simulink model "controller_template_vTST"  (Simulink 7.8)
settings: Solver=ode45  SolverMode=SingleTasking  StartTime=0.0  StopTime=20  FixedStep=Ts  RelTol=1e-3
PreLoadFcn:
  | load_waypoints
values from neighbouring files (symbols this model uses):
  Aff_pitch = [0.764669359834 -6.55628329998 -0.0099932514458 -0.411590904828 0.0133529191446 -0.0326334422872 -8.8646944178e-05 -0.00470014240893 0 0 1 0 ... (16 elements, 4x4)]    [kostas_malakies.mat]    (also in kostas_malakies2.mat)
  Aff_roll = [0.825180563081 -6.10606264808 -0.00763580464276 -0.367448917026 0.0145694646817 0.0253169520582 -6.457583527e-05 -0.00409059128644 0 0 1 0 ... (16 elements, 4x4)]    [kostas_malakies.mat]    (also in kostas_malakies2.mat; main_last.m = [Aff_roll,zeros(size(Aff_roll,1),1);zeros(1,size(Aff_roll,1))
  Aff_yaw = 0.520554464036    [kostas_malakies.mat]    (also in kostas_malakies2.mat; main.m = sysfd_yaw.a; main_last.m = sysfd_yaw.a)
  Bff_pitch = [0.235330640166  0; 6.55628329998  0; -0.000567656018985  0; -0.0435256495914  0]    [kostas_malakies.mat]    (also in kostas_malakies2.mat)
  Bff_roll = [0.174819436919  0; 6.10606264808  0; -0.000299760068643  0; -0.0270637325616  0]    [kostas_malakies.mat]    (also in kostas_malakies2.mat; main_last.m = [Bff_roll;zeros(1,size(Bff_roll,2))])
  Bff_yaw = 0.479445535964    [kostas_malakies.mat]    (also in kostas_malakies2.mat; main.m = sysfd_yaw.b; main_last.m = sysfd_yaw.b)
  Fi_XdirFF = [-0.447351940284 0 0 -1.28434394361 -4.04417159595 -1.80654990505 -1.28434394361 1 -4.04417159595 -1.80654990505 1 0 ... (536 elements, 134x4)]    [kostas_malakies.mat]    (also in kostas_malakies2.mat; matlab.mat = [-1.62441280603 -1.28434394361 -1.7723315065 -1.66810627541 )
  Fi_Yaw = [-1.14619813144 0 0]    [kostas_malakies.mat]    (also in kostas_malakies2.mat; matlab.mat = -0.284754025426)
  Fi_Ydir = [-0.466308586531 2.22044604925e-16 2.22044604925e-16 -1.46518332723 -4.54395337171 -2.00318743375 -1.46518332723 1 -4.54395337171 -2.00318743375 1 2.22044604925e-16 ... (536 elements, 134x4)]    [kostas_malakies.mat]    (also in kostas_malakies2.mat = [-0.521298425559 -2.64128186917 -15.6565978667 -8.2066553194; matlab.mat = [1 -1.9173235349 -1.46518332723 1 1 1 1 1 -1.98764774833 -1.)
  Fi_Zdir = [0 -1.80359099426e-16 0 1.4149586889 0 0 2.30859647265e-14 -5.77149118162e-15 0 0 0 0 ... (54 elements, 27x2)]    [kostas_malakies.mat]    (also in kostas_malakies2.mat = [4.30976351396 0 4.73307471514 3.80948040666 0 0 0 0.5468933; matlab.mat = [0 -9.51943523339e-14 0 1.99761158231 0 1.18992940417e-14 0 )
  g = 9.8065    [kostas_malakies.mat]    (also in kostas_malakies2.mat; load_PMModel.m = 9.81; main.m; main_last.m)
  Gi_XdirFF = [0 0.27 -0.27 0.478341621792 -6.42962779272 -1.98615606962 -0.478341621792 -0.373552567526 6.42962779272 1.98615606962 0.373552567526 0.27 ... (134 elements, 134x1)]    [kostas_malakies.mat]    (also in kostas_malakies2.mat; matlab.mat = [3.88578058619e-16 0.478341621792 -0.139455879222 -0.1159311)
  Gi_Yaw = [4.4408920985e-16 -3.14159265359 3.14159265359]    [kostas_malakies.mat]    (also in kostas_malakies2.mat = [-4.4408920985e-16 -3.14159265359 3.14159265359]; matlab.mat = 4.4408920985e-16)
  Gi_Ydir = [-2.77555756156e-16 0.27 -0.27 0.516209388722 7.06668201156 2.10835273651 -0.516209388722 -0.383863816771 -7.06668201156 -2.10835273651 0.383863816771 0.27 ... (134 elements, 134x1)]    [kostas_malakies.mat]    (also in kostas_malakies2.mat = [1.11022302463e-16 0.765579126644 531.260413192 11.754237275; matlab.mat = [0.383863816771 -0.133207088705 0.516209388722 0.38386381677)
  Gi_Zdir = [-1 -1 -1 2.22044604925e-16 -1 -1 -1 -1 1 -1 -1 -1 ... (27 elements, 27x1)]    [kostas_malakies.mat]    (also in kostas_malakies2.mat = [0.174387892495 -1 0.368373831608 3.33066907388e-16 -1 -1 -1; matlab.mat = [-2 -2 -2 1.11022302463e-15 -2 -2 -2 2 -2 -2 -2 2 ... (21 el)
  Hn_XdirFF = [-0.618529611748 0.618529611748 0.827215259158 -0.512155371354 -0.650909395739 -0.827215259158 0.930717154057 0.512155371354 0.650909395739 -0.930717154057 -1 0 ... (4464 elements, 1116x4)]    [kostas_malakies.mat]    (also in kostas_malakies2.mat; matlab.mat = [1 -0.136019433325 -0.405248495598 -0.339279056031 0 -1 0.13)
  Hn_Yaw = [1 -1 -1 1 1 -1]    [kostas_malakies.mat]    (also in kostas_malakies2.mat; matlab.mat = [1 -1])
  Hn_Ydir = [-0.642151612842 0.642151612842 0.873369621238 0.521434628645 0.668917219747 -0.873369621238 0.934789012395 -0.521434628645 -0.668917219747 -0.934789012395 -1 0 ... (4532 elements, 1133x4)]    [kostas_malakies.mat]    (also in kostas_malakies2.mat = [0.972602710123 0.0284063109089 0.559530157965 0.73050130567; matlab.mat = [0.711566553558 0.999813894311 -0.735660470031 0 0 0.5471922)
  Hn_Zdir = [-0.560552458797 -0.996815278536 -0.988320507921 0.666673243042 -1 0 -0.421994354267 -0.987440631917 -0.973284290019 -0.956170964903 -0.936236606521 0.560552458797 ... (224 elements, 112x2)]    [kostas_malakies.mat]    (also in kostas_malakies2.mat = [-0.781813705838 -0.712499731132 0.751798766698 0 -0.7286973; matlab.mat = [1 -1 -0.996815278536 -0.990718937584 -0.276007160242 0.3840)
  Kn_XdirFF = [0.373314565409 0.373314565409 0.472754204418 0.915522246067 0.951154784392 0.472754204418 0.240212330437 0.915522246067 0.951154784392 0.240212330437 0.2094 2 ... (1116 elements, 1116x1)]    [kostas_malakies.mat]    (also in kostas_malakies2.mat; matlab.mat = [0.2094 0.19132523886 0.382063154155 0.900203176458 2 0.2094)
  Kn_Yaw = [2.74088097634 2.74088097634 -2.74088097634 3.14159265359 -2.74088097634 3.14159265359]    [kostas_malakies.mat]    (also in kostas_malakies2.mat; matlab.mat = [0.0873 0.0873])
  Kn_Ydir = [0.371815875743 0.371815875743 0.451349483511 0.90366201682 0.917647772499 0.451349483511 0.24471770913 0.90366201682 0.917647772499 0.24471770913 0.2094 2 ... (1133 elements, 1133x1)]    [kostas_malakies.mat]    (also in kostas_malakies2.mat = [0.351231202126 0.997082913977 0.855763802521 0.792250278627; matlab.mat = [-0.126119149197 0.0536759032179 0.37354703421 2 2 -0.239682)
  Kn_Zdir = [0.727672356179 1.00172267683 1.00656919451 -0.471160923828 1 1 1.18526984431 1.00688561667 1.01272393898 1.01603878926 1.01572683497 -0.727672356179 ... (112 elements, 112x1)]    [kostas_malakies.mat]    (also in kostas_malakies2.mat = [0.21304012328 0.326509029469 -0.262060822346 1 0.301409884 ; matlab.mat = [1 1 1.00663007512 1.02122194908 0.632590992205 -0.384463644)
  Nc_XdirFF = [18 15 15 11 9 7 11 14 9 7 14 8 ... (134 elements, 134x1)]    [kostas_malakies.mat]    (also in kostas_malakies2.mat; matlab.mat = [14 8 7 10 8 7 10 12 10 10 12 11 ... (107 elements, 107x1)])
  Nc_Yaw = [2 2 2]    [kostas_malakies.mat]    (also in kostas_malakies2.mat; matlab.mat = 2)
  Nc_Ydir = [18 16 16 10 9 7 10 14 9 7 14 8 ... (134 elements, 134x1)]    [kostas_malakies.mat]    (also in kostas_malakies2.mat = [22 12 6 9 9 5 12 13 6 9 9 5 ... (171 elements, 171x1)]; matlab.mat = [11 8 12 15 7 9 10 13 10 14 12 7 ... (104 elements, 104x1)])
  Nc_Zdir = [6 7 3 6 3 4 4 3 6 5 3 4 ... (27 elements, 27x1)]    [kostas_malakies.mat]    (also in kostas_malakies2.mat = [4 4 3 12 5 4 3 3 4 3 3 4 ... (93 elements, 93x1)]; matlab.mat = [6 3 7 4 4 3 4 6 3 5 3 3 ... (21 elements, 21x1)])
  pitch_cmd2pitch_1stOrd = 1.42468924998    [kostas_malakies.mat]    (also in kostas_malakies2.mat)
  roll_cmd2roll_1stOrd = 1.38101661575    [kostas_malakies.mat]    (also in kostas_malakies2.mat)
  thrust_cmd2thrust_0thOrd = 0.876575459522    [kostas_malakies.mat]    (also in kostas_malakies2.mat)
  THRUST_CMD_GAIN = -0.0835    [kostas_malakies.mat]    (also in kostas_malakies2.mat; load_PMModel.m)
  Ts = 0.02    [kostas_malakies.mat]    (also in kostas_malakies2.mat; main.m; main_last.m; matlab.mat = 0.08)
  yaw_cmd2yaw_1stOrd = 2.01792090263    [kostas_malakies.mat]    (also in kostas_malakies2.mat)
  z = [-0.93079906702 -0.933865725994 -0.937557637691 -0.939011216164 -0.94143640995 -0.944628417492 -0.947235524654 -0.949601888657 -0.952827751637 -0.9567258358 -0.958320975304 -0.960991024971 ... (7988 elements, 7988x1)]    [kostas_malakies2.mat]    (also in plotDataTest.m = simout_data.signals.values(:,11))
libraries: simulink x6, Hquad_control_LIB_MPC x5
(part 1 of 2)
settings Model: Creator=janosch  LastModifiedBy=burrimi
settings DataIOCC: SaveOutput=off  SaveTime=off
settings OptimizationCC: OptimizeModelRefInitCode=on  LifeSpan=Inf
settings DebuggingCC: ParameterPrecisionLossMsg=none
settings HardwareCC: ProdIntDivRoundTo=Zero  ProdEndianess=LittleEndian  ProdHWDeviceType=Intel Pentium
settings RTWCC: SystemTargetFile=ert.tlc  TemplateMakefile=ert_default_tmf  Description=Embedded Coder  ProcessScript=ert_make_rtw_hook  CustomHeaderCode=#include <math.h>  TargetLang=C++  RTWCompilerOptimization=On
settings CodeAppCC: IgnoreCustomStorageClasses=off
settings ERTTargetCC: MultiwordLength=2048  GenerateSampleERTMain=on  ExtMode=on  ERTCustomFileTemplate=example_file_process.tlc  ConvertIfToSwitch=off  SuppressUnreachableDefaultCases=off

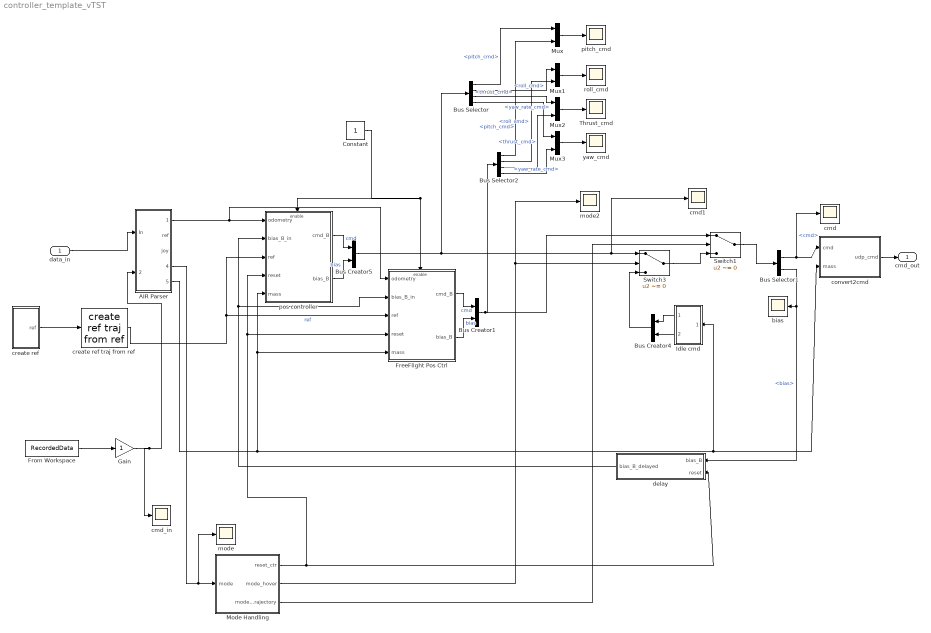
== system controller_template_vTST ==
  data_in : Inport  OutDataTypeStr=single  PortDimensions=30
  AIR Parser : Subsystem
  Bus Creator1 : BusCreator  Inputs=2
  Bus Creator4 : BusCreator  Inputs=2
  Bus Creator5 : BusCreator  Inputs=2
  Bus Selector : BusSelector  OutputSignals=cmd.pitch_cmd,cmd.roll_cmd,cmd.thrust_cmd,cmd.yaw_rate_cmd
  Bus Selector1 : BusSelector  OutputSignals=cmd,bias
  Bus Selector2 : BusSelector  OutputSignals=cmd.pitch_cmd,cmd.roll_cmd,cmd.thrust_cmd,cmd.yaw_rate_cmd
  Constant : Constant
  FreeFlight Pos Ctrl : Subsystem  AncestorBlock=Hquad_control_LIB_MPC/pos controller
  From Workspace : FromWorkspace  VariableName=RecordedData  SampleTime=0
  Gain : Gain  SampleTime=Ts
  Idle cmd : Subsystem
  Mode Handling : Subsystem
  Mux{,1..3} (4 alike) : Mux  Inputs=2
  Switch1 : Switch  Criteria=u2 ~= 0
  Switch3 : Switch  Criteria=u2 ~= 0
  Thrust_cmd : Scope
      settings: YMin=-1.3  YMax=0.1  SaveName=ScopeData18
  bias : Scope
      settings: TickLabels=on  TimeRange=40  YMin=-0.3  YMax=0.075  SaveName=ScopeData9
  cmd : Scope
      settings: YMin=-0.5  YMax=7  SaveName=ScopeData4
  cmd1 : Scope
      settings: YMin=-0.5  YMax=7  SaveName=ScopeData15
  cmd_in : Scope
      settings: YMin=-0.05  YMax=1.05  SaveName=ScopeData16
  convert2cmd : Subsystem
  create ref : Subsystem  AncestorBlock=Hquad_control_LIB_LQRI/create ref
  create ref traj from ref : Hquad_control_LIB_MPC/create ref traj from ref
  delay : Subsystem
  mode : Scope
      settings: YMin=0  YMax=6  SaveName=ScopeData6
  mode2 : Scope
      settings: YMin=0  YMax=6  SaveName=ScopeData14
  pitch_cmd : Scope
      settings: YMin=-0.375  YMax=0.1  SaveName=ScopeData13
  pos controller : Subsystem  AncestorBlock=Hquad_control_LIB_MPC/pos controller
  roll_cmd : Scope
      settings: YMin=-0.275  YMax=0.125  SaveName=ScopeData17
  yaw_cmd : Scope
      settings: YMin=-0.025  YMax=0.475  SaveName=ScopeData19
  cmd_out : Outport  PortDimensions=4
  wires:
  Mode Handling/1(reset_ctr) -> delay/2(reset), pos controller/4(reset), FreeFlight Pos Ctrl/4(reset)
  Mode Handling/2(mode_hover) -> Switch3/2, mode2/1
  AIR Parser/4(mode) -> mode/1, Mode Handling/1(mode)
  Bus Creator5/1 -> Switch3/1, cmd1/1, Bus Selector/1
  pos controller/1(cmd_B) -> Bus Creator5/1  "cmd"
  pos controller/2(bias_B) -> Bus Creator5/2  "bias"
  Bus Selector1/1 -> convert2cmd/1(cmd), cmd/1  "<cmd>"
  Bus Selector1/2 -> bias/1, delay/1(bias_B)  "<bias>"
  delay/1(bias_B_delayed) -> pos controller/2(bias_B_in), FreeFlight Pos Ctrl/2(bias_B_in)
  convert2cmd/1(udp_cmd) -> cmd_out/1
  data_in/1 -> AIR Parser/1(In)
  Idle cmd/1(cmd) -> Bus Creator4/1
  Idle cmd/2(bias) -> Bus Creator4/2
  Bus Creator4/1 -> Switch3/3
  AIR Parser/1(odometry) -> pos controller/1(odometry), FreeFlight Pos Ctrl/1(odometry)
  Switch3/1 -> Switch1/3
  Switch1/1 -> Bus Selector1/1
  Mode Handling/3(mode_trajectory) -> Switch1/2
  AIR Parser/5(mass) -> Idle cmd/1(mass), convert2cmd/2(mass), pos controller/5(mass), FreeFlight Pos Ctrl/5(mass)
  create ref traj from ref/1 -> pos controller/3(ref), FreeFlight Pos Ctrl/3(ref)  "ref"
  Bus Creator1/1 -> Switch1/1, Bus Selector2/1
  FreeFlight Pos Ctrl/1(cmd_B) -> Bus Creator1/1  "cmd"
  FreeFlight Pos Ctrl/2(bias_B) -> Bus Creator1/2  "bias"
  From Workspace/1 -> Gain/1
  Gain/1 -> AIR Parser/2(Recorded), cmd_in/1
  Constant/1 -> pos controller/Enable, FreeFlight Pos Ctrl/Enable
  Bus Selector/1 -> Mux/1  "<pitch_cmd>"
  Mux/1 -> pitch_cmd/1
  create ref/1(ref) -> create ref traj from ref/1
  Mux1/1 -> roll_cmd/1
  Mux2/1 -> Thrust_cmd/1
  Mux3/1 -> yaw_cmd/1
  Bus Selector/2 -> Mux1/1  "<roll_cmd>"
  Bus Selector/3 -> Mux2/1  "<thrust_cmd>"
  Bus Selector/4 -> Mux3/1  "<yaw_rate_cmd>"
  Bus Selector2/2 -> Mux1/2  "<roll_cmd>"
  Bus Selector2/3 -> Mux2/2  "<thrust_cmd>"
  Bus Selector2/4 -> Mux3/2  "<yaw_rate_cmd>"
  Bus Selector2/1 -> Mux/2  "<pitch_cmd>"

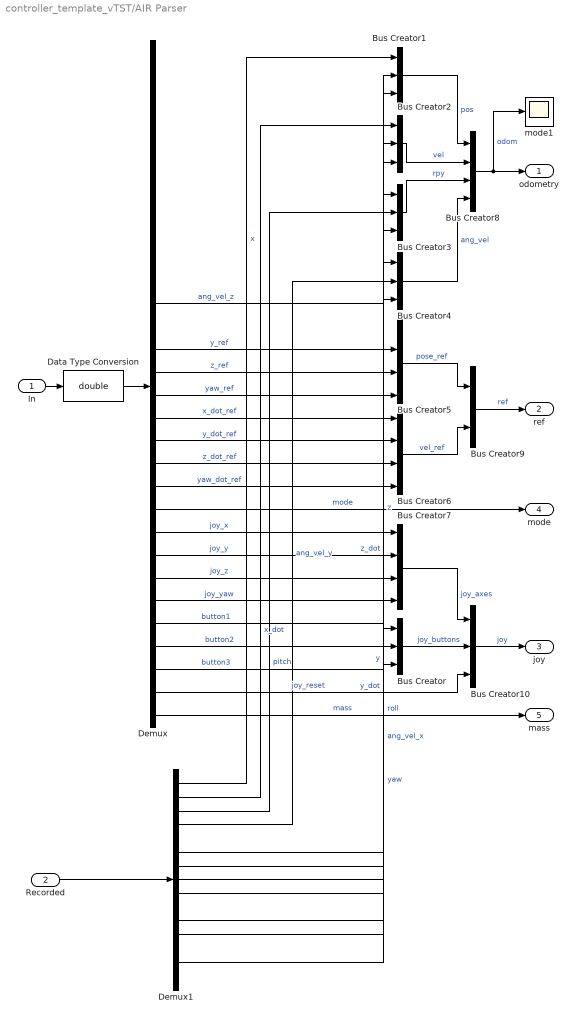
== system controller_template_vTST/AIR Parser ==
  In : Inport
  Recorded : Inport  Port=2
  Bus Creator{,1..4,10} (6 alike) : BusCreator  Inputs=3
  Bus Creator{5..8} (4 alike) : BusCreator
  Bus Creator9 : BusCreator  Inputs=2
  Data Type Conversion : DataTypeConversion  OutDataTypeStr=double
  Demux : Demux  Outputs=30
  Demux1 : Demux  Outputs=15
  mode1 : Scope
      settings: YMin=0  YMax=6  SaveName=ScopeData7
  odometry : Outport
  ref : Outport  Port=2
  joy : Outport  Port=3
  mode : Outport  Port=4
  mass : Outport  Port=5
  wires:
  In/1 -> Data Type Conversion/1
  Data Type Conversion/1 -> Demux/1
  Demux/15 -> Bus Creator5/3  "z_ref"
  Demux/14 -> Bus Creator5/2  "y_ref"
  Demux/16 -> Bus Creator5/4  "yaw_ref"
  Demux/19 -> Bus Creator6/3  "z_dot_ref"
  Demux/18 -> Bus Creator6/2  "y_dot_ref"
  Demux/17 -> Bus Creator6/1  "x_dot_ref"
  Demux/20 -> Bus Creator6/4  "yaw_dot_ref"
  Demux/12 -> Bus Creator4/3  "ang_vel_z"
  Demux/21 -> mode/1  "mode"
  Bus Creator5/1 -> Bus Creator9/1  "pose_ref"
  Bus Creator6/1 -> Bus Creator9/2  "vel_ref"
  Demux/22 -> Bus Creator7/1  "joy_x"
  Demux/23 -> Bus Creator7/2  "joy_y"
  Demux/24 -> Bus Creator7/3  "joy_z"
  Demux/25 -> Bus Creator7/4  "joy_yaw"
  Bus Creator7/1 -> Bus Creator10/1  "joy_axes"
  Demux/26 -> Bus Creator/1  "button1"
  Demux/28 -> Bus Creator/3  "button3"
  Demux/27 -> Bus Creator/2  "button2"
  Bus Creator/1 -> Bus Creator10/2  "joy_buttons"
  Bus Creator4/1 -> Bus Creator8/4  "ang_vel"
  Bus Creator3/1 -> Bus Creator8/3  "rpy"
  Bus Creator2/1 -> Bus Creator8/2  "vel"
  Bus Creator1/1 -> Bus Creator8/1  "pos"
  Demux/29 -> Bus Creator10/3  "joy_reset"
  Bus Creator10/1 -> joy/1  "joy"
  Bus Creator9/1 -> ref/1  "ref"
  Bus Creator8/1 -> odometry/1, mode1/1  "odom"
  Demux/30 -> mass/1  "mass"
  Recorded/1 -> Demux1/1
  Demux1/1 -> Bus Creator1/1  "x"
  Demux1/2 -> Bus Creator2/1  "x_dot"
  Demux1/3 -> Bus Creator3/2  "pitch"
  Demux1/4 -> Bus Creator4/2  "ang_vel_y"
  Demux1/7 -> Bus Creator2/2  "y_dot"
  Demux1/8 -> Bus Creator3/1  "roll"
  Demux1/9 -> Bus Creator4/1  "ang_vel_x"
  Demux1/12 -> Bus Creator2/3  "z_dot"
  Demux1/6 -> Bus Creator1/2  "y"
  Demux1/11 -> Bus Creator1/3  "z"
  Demux1/14 -> Bus Creator3/3  "yaw"

== system controller_template_vTST/FreeFlight Pos Ctrl ==
  odometry : Inport
  bias_B_in : Inport  Port=2
  ref : Inport  Port=3
  reset : Inport  Port=4
  mass : Inport  Port=5
  Enable : EnablePort  StatesWhenEnabling=reset
  MAIN CONTROL LOOP1 : Subsystem  Priority=2  AncestorBlock=Hquad_control_LIB_MPC/MAIN CONTROL LOOP  TreatAsAtomicUnit=on
  get ref from vector : Hquad_control_LIB_MPC/pos controller/get ref from vector
  rotate to world frame : Hquad_control_LIB_MPC/rotate to world frame  Priority=1
  view & log signals : Subsystem  AncestorBlock=Hquad_control_LIB_MPC/view & log signals
  cmd_B : Outport
  bias_B : Outport  Port=2
  wires:
  mass/1 -> MAIN CONTROL LOOP1/5(mass)
  bias_B_in/1 -> rotate to world frame/2
  rotate to world frame/2 -> MAIN CONTROL LOOP1/2(bias_W)
  rotate to world frame/1 -> MAIN CONTROL LOOP1/1(odometry), view & log signals/1(odometry)
  ref/1 -> get ref from vector/1
  reset/1 -> MAIN CONTROL LOOP1/4(reset)
  odometry/1 -> rotate to world frame/1
  get ref from vector/1 -> MAIN CONTROL LOOP1/3(ref), view & log signals/2(ref)
  MAIN CONTROL LOOP1/1(cmd_W) -> view & log signals/3(cmd), cmd_B/1
  MAIN CONTROL LOOP1/2(bias_W_out) -> view & log signals/4(bias), bias_B/1

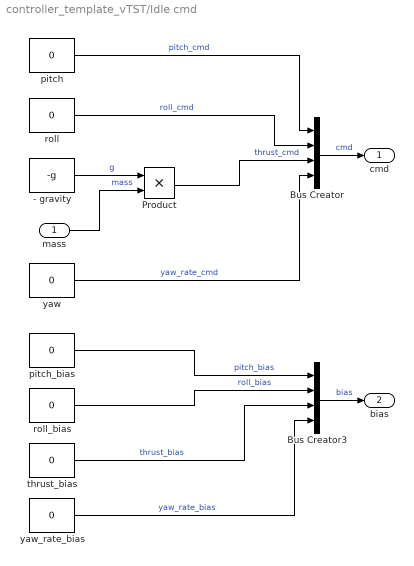
== system controller_template_vTST/Idle cmd ==
  mass : Inport  OutDataTypeStr=double
  - gravity : Constant  Value=-g
  Bus Creator : BusCreator
  Bus Creator3 : BusCreator
  Product : Product  RndMeth=Zero
  pitch : Constant  Value=0
  pitch_bias : Constant  Value=0
  roll : Constant  Value=0
  roll_bias : Constant  Value=0
  thrust_bias : Constant  Value=0
  yaw : Constant  Value=0
  yaw_rate_bias : Constant  Value=0
  cmd : Outport
  bias : Outport  Port=2
  wires:
  roll/1 -> Bus Creator/2  "roll_cmd"
  pitch/1 -> Bus Creator/1  "pitch_cmd"
  Bus Creator/1 -> cmd/1  "cmd"
  yaw/1 -> Bus Creator/4  "yaw_rate_cmd"
  pitch_bias/1 -> Bus Creator3/1  "pitch_bias"
  roll_bias/1 -> Bus Creator3/2  "roll_bias"
  thrust_bias/1 -> Bus Creator3/3  "thrust_bias"
  yaw_rate_bias/1 -> Bus Creator3/4  "yaw_rate_bias"
  Bus Creator3/1 -> bias/1  "bias"
  - gravity/1 -> Product/1  "g"
  Product/1 -> Bus Creator/3  "thrust_cmd"
  mass/1 -> Product/2  "mass"

== system controller_template_vTST/Mode Handling ==
  mode : Inport
  Constant1 : Constant
  Constant2 : Constant  Value=0
  Multiport Switch : MultiPortSwitch  DataPortOrder=Specify indices  Inputs=2  DataPortIndices={[1,2,3],0}  zeroidx=off
  Multiport Switch1 : MultiPortSwitch  DataPortOrder=Specify indices  Inputs=2  DataPortIndices={[10],0}  zeroidx=off
  Multiport Switch2 : MultiPortSwitch  DataPortOrder=Specify indices  Inputs=2  DataPortIndices={[4],0}  zeroidx=off
  reset_ctr : Outport
  mode_hover : Outport  Port=2
  mode_trajectory : Outport  Port=3
  wires:
  Constant1/1 -> Multiport Switch/2, Multiport Switch1/2, Multiport Switch2/2
  Constant2/1 -> Multiport Switch/3, Multiport Switch1/3, Multiport Switch2/3
  Multiport Switch1/1 -> reset_ctr/1
  mode/1 -> Multiport Switch/1, Multiport Switch1/1, Multiport Switch2/1
  Multiport Switch/1 -> mode_hover/1
  Multiport Switch2/1 -> mode_trajectory/1

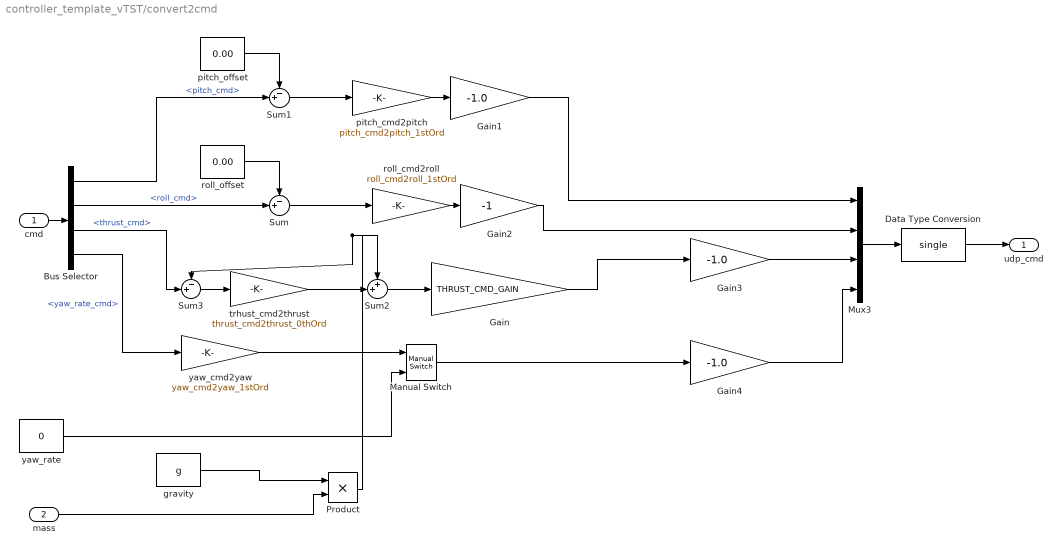
== system controller_template_vTST/convert2cmd ==
  cmd : Inport
  mass : Inport  Port=2
  Bus Selector : BusSelector  OutputSignals=pitch_cmd,roll_cmd,thrust_cmd,yaw_rate_cmd
  Data Type Conversion : DataTypeConversion  OutDataTypeStr=single
  Gain : Gain  Gain=THRUST_CMD_GAIN
  Gain1 : Gain  Gain=-1.0
  Gain2 : Gain  Gain=-1
  Gain3 : Gain  Gain=-1.0
  Gain4 : Gain  Gain=-1.0
  Manual Switch : simulink/Signal Routing/Manual Switch  sw=1  action=0  varsize=off
  Mux3 : Mux
  Product : Product  RndMeth=Zero
  Sum : Sum  Inputs=-+|
  Sum1 : Sum  Inputs=-+|
  Sum2 : Sum  Inputs=++|
  Sum3 : Sum  Inputs=-+|
  gravity : Constant  Value=g
  pitch_cmd2pitch : Gain  Gain=pitch_cmd2pitch_1stOrd
  pitch_offset : Constant  Value=0.00
  roll_cmd2roll : Gain  Gain=roll_cmd2roll_1stOrd
  roll_offset : Constant  Value=0.00
  trhust_cmd2thrust : Gain  Gain=thrust_cmd2thrust_0thOrd
  yaw_cmd2yaw : Gain  Gain=yaw_cmd2yaw_1stOrd
  yaw_rate : Constant  Value=0
  udp_cmd : Outport
  wires:
  pitch_cmd2pitch/1 -> Gain1/1
  Bus Selector/2 -> Sum/2  "<roll_cmd>"
  Sum/1 -> roll_cmd2roll/1
  roll_offset/1 -> Sum/1
  Gain4/1 -> Mux3/4
  Gain3/1 -> Mux3/3
  Gain2/1 -> Mux3/2
  Gain/1 -> Gain3/1
  Gain1/1 -> Mux3/1
  pitch_offset/1 -> Sum1/1
  Sum1/1 -> pitch_cmd2pitch/1
  Mux3/1 -> Data Type Conversion/1
  Data Type Conversion/1 -> udp_cmd/1
  Product/1 -> Sum2/1, Sum3/1
  Sum2/1 -> Gain/1
  Manual Switch/1 -> Gain4/1
  yaw_rate/1 -> Manual Switch/2
  cmd/1 -> Bus Selector/1
  Bus Selector/1 -> Sum1/2  "<pitch_cmd>"
  yaw_cmd2yaw/1 -> Manual Switch/1
  trhust_cmd2thrust/1 -> Sum2/2
  roll_cmd2roll/1 -> Gain2/1
  Bus Selector/3 -> Sum3/2  "<thrust_cmd>"
  Sum3/1 -> trhust_cmd2thrust/1
  Bus Selector/4 -> yaw_cmd2yaw/1  "<yaw_rate_cmd>"
  gravity/1 -> Product/1
  mass/1 -> Product/2

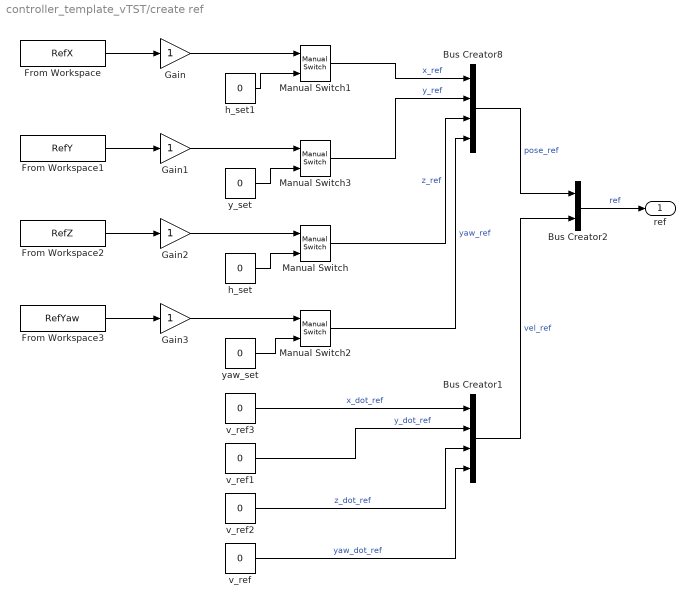
== system controller_template_vTST/create ref ==
  Bus Creator1 : BusCreator
  Bus Creator2 : BusCreator  Inputs=2
  Bus Creator8 : BusCreator
  From Workspace : FromWorkspace  VariableName=RefX  SampleTime=0
  From Workspace1 : FromWorkspace  VariableName=RefY  SampleTime=0
  From Workspace2 : FromWorkspace  VariableName=RefZ  SampleTime=0
  From Workspace3 : FromWorkspace  VariableName=RefYaw  SampleTime=0
  Gain{,1..3} (4 alike) : Gain  SampleTime=Ts
  Manual Switch{,1..3} (4 alike) : simulink/Signal Routing/Manual Switch  sw=1  action=0  varsize=off
  h_set : Constant  Value=0  OutDataTypeStr=double  SampleTime=-1
  h_set1 : Constant  Value=0  OutDataTypeStr=double  SampleTime=-1
  v_ref{,1..3} (4 alike) : Constant  Value=0  OutDataTypeStr=double  SampleTime=-1
  y_set : Constant  Value=0  OutDataTypeStr=double  SampleTime=-1
  "yaw_set  " : Constant  Value=0  OutDataTypeStr=double  SampleTime=-1
  ref : Outport
  wires:
  Gain3/1 -> Manual Switch2/1
  "yaw_set  "/1 -> Manual Switch2/2
  h_set/1 -> Manual Switch/2
  Gain2/1 -> Manual Switch/1
  Gain1/1 -> Manual Switch3/1
  y_set/1 -> Manual Switch3/2
  h_set1/1 -> Manual Switch1/2
  Bus Creator2/1 -> ref/1  "ref"
  Bus Creator8/1 -> Bus Creator2/1  "pose_ref"
  Bus Creator1/1 -> Bus Creator2/2  "vel_ref"
  Manual Switch1/1 -> Bus Creator8/1  "x_ref"
  Manual Switch3/1 -> Bus Creator8/2  "y_ref"
  Manual Switch2/1 -> Bus Creator8/4  "yaw_ref"
  Manual Switch/1 -> Bus Creator8/3  "z_ref"
  v_ref/1 -> Bus Creator1/4  "yaw_dot_ref"
  v_ref3/1 -> Bus Creator1/1  "x_dot_ref"
  v_ref1/1 -> Bus Creator1/2  "y_dot_ref"
  v_ref2/1 -> Bus Creator1/3  "z_dot_ref"
  Gain/1 -> Manual Switch1/1
  From Workspace/1 -> Gain/1
  From Workspace1/1 -> Gain1/1
  From Workspace2/1 -> Gain2/1
  From Workspace3/1 -> Gain3/1

== system controller_template_vTST/delay ==
  bias_B : Inport
  reset : Inport  Port=2
  Bus Creator1 : BusCreator
  Demux1 : Demux
  delay bias : simulink/Additional Math & Discrete/Additional Discrete/Unit Delay Resettable  vinit=0.0  tsamp=-1
  bias_B_delayed : Outport
  wires:
  Demux1/1 -> Bus Creator1/1  "pitch_bias"
  Demux1/2 -> Bus Creator1/2  "roll_bias"
  Demux1/3 -> Bus Creator1/3  "thrust_bias"
  Demux1/4 -> Bus Creator1/4  "yaw_rate_bias"
  delay bias/1 -> Demux1/1
  bias_B/1 -> delay bias/1
  reset/1 -> delay bias/2
  Bus Creator1/1 -> bias_B_delayed/1

== system controller_template_vTST/pos controller ==
  odometry : Inport
  bias_B_in : Inport  Port=2
  ref : Inport  Port=3
  reset : Inport  Port=4
  mass : Inport  Port=5
  Enable : EnablePort  StatesWhenEnabling=reset
  MAIN CONTROL LOOP1 : Hquad_control_LIB_MPC/MAIN CONTROL LOOP  Priority=2
  get ref from vector : Subsystem
  mode1 : Scope
      settings: YMin=0  YMax=6  SaveName=ScopeData12
  rotate to world frame : Hquad_control_LIB_MPC/rotate to world frame  Priority=1
  view & log signals : Subsystem  AncestorBlock=Hquad_control_LIB_MPC/view & log signals
  cmd_B : Outport
  bias_B : Outport  Port=2
  wires:
  MAIN CONTROL LOOP1/1 -> view & log signals/3(cmd), cmd_B/1
  odometry/1 -> rotate to world frame/1, view & log signals/1(odometry)
  reset/1 -> MAIN CONTROL LOOP1/4
  ref/1 -> get ref from vector/1(X_ref), MAIN CONTROL LOOP1/3
  get ref from vector/1(ref) -> view & log signals/2(ref), mode1/1
  rotate to world frame/1 -> MAIN CONTROL LOOP1/1
  MAIN CONTROL LOOP1/2 -> view & log signals/4(bias), bias_B/1
  rotate to world frame/2 -> MAIN CONTROL LOOP1/2
  bias_B_in/1 -> rotate to world frame/2
  mass/1 -> MAIN CONTROL LOOP1/5

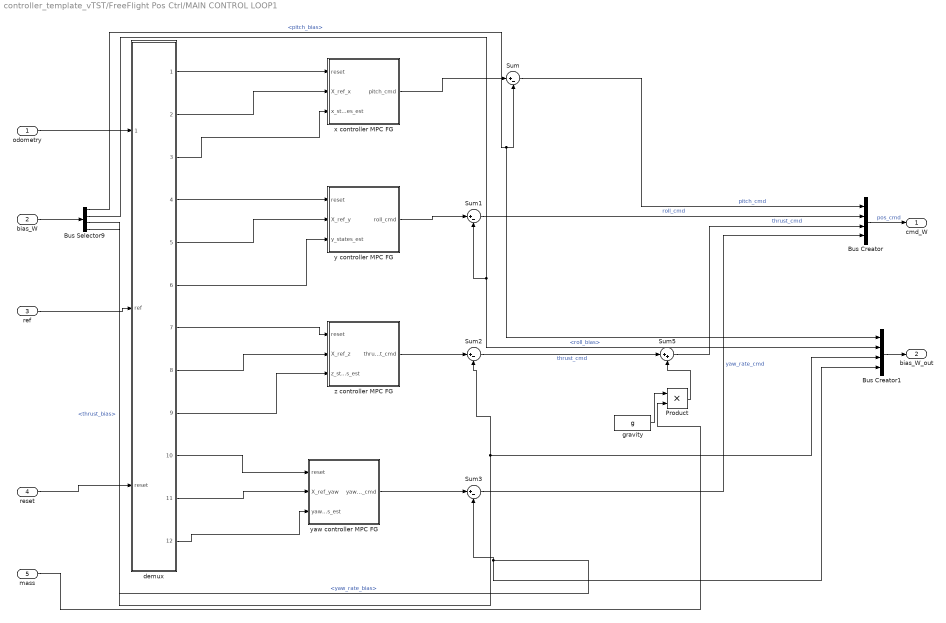
== system controller_template_vTST/FreeFlight Pos Ctrl/MAIN CONTROL LOOP1 ==
  odometry : Inport
  bias_W : Inport  Port=2
  ref : Inport  Port=3
  reset : Inport  Port=4
  mass : Inport  Port=5
  Bus Creator : BusCreator
  Bus Creator1 : BusCreator
  Bus Selector9 : BusSelector  OutputSignals=pitch_bias,roll_bias,thrust_bias,yaw_rate_bias
  Product : Product  RndMeth=Zero
  Sum{,1..3} (4 alike) : Sum  Inputs=|+-
  Sum5 : Sum  Inputs=|++
  demux : Subsystem
  gravity : Constant  Value=g
  "x controller MPC FG  " : Subsystem  AncestorBlock=Hquad_control_LIB_MPC/x controller MPC FG
  y controller MPC FG : Subsystem  AncestorBlock=Hquad_control_LIB_MPC/y controller MPC FG
  yaw controller MPC FG : Subsystem  AncestorBlock=Hquad_control_LIB_MPC/yaw controller MPC FG
  z controller MPC FG : Subsystem  AncestorBlock=Hquad_control_LIB_MPC/z controller MPC FG
  cmd_W : Outport
  bias_W_out : Outport  Port=2
  wires:
  Bus Selector9/4 -> Sum3/2, Bus Creator1/4  "<yaw_rate_bias>"
  Sum3/1 -> Bus Creator/4  "yaw_rate_cmd"
  Bus Selector9/3 -> Sum2/2, Bus Creator1/3  "<thrust_bias>"
  Bus Selector9/1 -> Sum/2, Bus Creator1/1  "<pitch_bias>"
  Bus Selector9/2 -> Bus Creator1/2, Sum1/2  "<roll_bias>"
  bias_W/1 -> Bus Selector9/1
  Sum5/1 -> Bus Creator/3  "thrust_cmd"
  Bus Creator1/1 -> bias_W_out/1
  Sum2/1 -> Sum5/1  "thrust_cmd"
  Sum1/1 -> Bus Creator/2  "roll_cmd"
  Sum/1 -> Bus Creator/1  "pitch_cmd"
  odometry/1 -> demux/1(odometry)
  ref/1 -> demux/2(ref)
  reset/1 -> demux/3(reset)
  demux/1(reset1) -> "x controller MPC FG  "/1(reset)
  demux/4(reset2) -> y controller MPC FG/1(reset)
  demux/7(reset3) -> z controller MPC FG/1(reset)
  demux/10(reset4) -> yaw controller MPC FG/1(reset)
  Bus Creator/1 -> cmd_W/1  "pos_cmd"
  mass/1 -> Product/2
  Product/1 -> Sum5/2
  gravity/1 -> Product/1
  "x controller MPC FG  "/1("pitch_cmd   ") -> Sum/1
  y controller MPC FG/1(roll_cmd) -> Sum1/1
  z controller MPC FG/1(thrust_cmd) -> Sum2/1
  yaw controller MPC FG/1(yaw_rate_cmd) -> Sum3/1
  demux/2(X_ref_x) -> "x controller MPC FG  "/2("X_ref_x  ")
  demux/3(x_states) -> "x controller MPC FG  "/3("x_states_est  ")
  demux/5(X_ref_y) -> y controller MPC FG/2("X_ref_y  ")
  demux/8(X_ref_z) -> z controller MPC FG/2(X_ref_z)
  demux/9(z_states) -> z controller MPC FG/3("z_states_est  ")
  demux/11(X_ref_yaw) -> yaw controller MPC FG/2(X_ref_yaw)
  demux/12(yaw_states) -> yaw controller MPC FG/3("yaw_states_est  ")
  demux/6(y_states) -> y controller MPC FG/3("y_states_est  ")

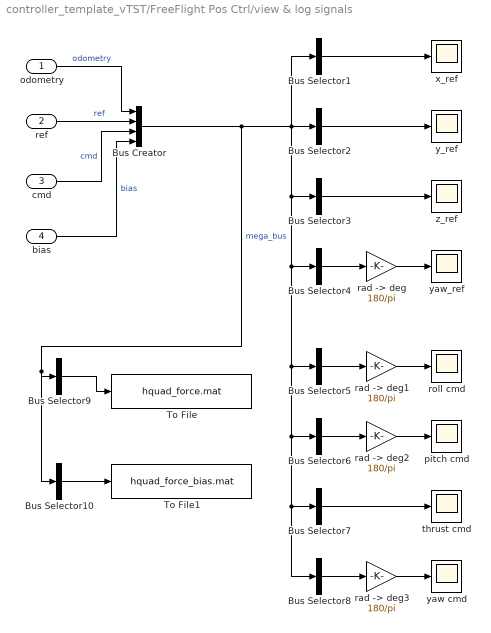
== system controller_template_vTST/FreeFlight Pos Ctrl/view & log signals ==
  odometry : Inport
  ref : Inport  Port=2
  cmd : Inport  Port=3
  bias : Inport  Port=4
  Bus Creator : BusCreator
  Bus Selector1 : BusSelector  OutputSignals=odometry.pos.x,odometry.vel.x_dot,ref.pose_ref.x_ref,ref.vel_ref.x_dot_ref  OutputAsBus=on
  Bus Selector10 : BusSelector  OutputSignals=bias.pitch_bias,bias.roll_bias,bias.thrust_bias,bias.yaw_rate_bias  OutputAsBus=on
  Bus Selector2 : BusSelector  OutputSignals=odometry.pos.y,odometry.vel.y_dot,ref.pose_ref.y_ref,ref.vel_ref.y_dot_ref  OutputAsBus=on
  Bus Selector3 : BusSelector  OutputSignals=odometry.pos.z,odometry.vel.z_dot,ref.pose_ref.z_ref,ref.vel_ref.z_dot_ref  OutputAsBus=on
  Bus Selector4 : BusSelector  OutputSignals=odometry.rpy.yaw,odometry.ang_vel.ang_vel_z,ref.pose_ref.yaw_ref,ref.vel_ref.yaw_dot_ref  OutputAsBus=on
  Bus Selector5 : BusSelector  OutputSignals=odometry.rpy.roll,odometry.ang_vel.ang_vel_x,cmd.roll_cmd  OutputAsBus=on
  Bus Selector6 : BusSelector  OutputSignals=odometry.rpy.pitch,odometry.ang_vel.ang_vel_y,cmd.pitch_cmd  OutputAsBus=on
  Bus Selector7 : BusSelector  OutputSignals=odometry.pos.z,ref.pose_ref.z_ref,cmd.thrust_cmd  OutputAsBus=on
  Bus Selector8 : BusSelector  OutputSignals=odometry.rpy.yaw,odometry.ang_vel.ang_vel_z,cmd.yaw_rate_cmd  OutputAsBus=on
  Bus Selector9 : BusSelector  OutputSignals=odometry.pos.x,odometry.vel.x_dot,odometry.rpy.pitch,ref.pose_ref.x_ref,cmd.pitch_cmd,odometry.pos.y,odometry.vel.y_dot,odometry.rpy.roll,ref.pose_ref.y_ref,cmd.roll_cmd,odometry.pos.z,odometry.vel.z_dot,ref.pose_ref.z_ref,cmd.thrust_cmd,odometry.rpy.yaw,odometry.ang_vel.ang_vel_z,ref.pose_ref.yaw_ref,cmd.yaw_rate_cmd  OutputAsBus=on
  To File : ToFile  Filename=hquad_force.mat  MatrixName=hquad_force
  To File1 : ToFile  Filename=hquad_force_bias.mat  MatrixName=hquad_force_bias
  pitch cmd : Scope
      settings: YMin=-15  YMax=15  SaveName=ScopeData2
  rad -> deg{,1..3} (4 alike) : Gain  Gain=180/pi
  roll cmd : Scope
      settings: YMin=-100  YMax=100
  thrust cmd : Scope
      settings: YMin=-3  YMax=3  SaveName=ScopeData11
  x_ref : Scope
      settings: YMin=-1.5  YMax=1.5  SaveName=ScopeData3
  y_ref : Scope
      settings: TimeRange=40  YMin=-0.75  YMax=2.75
  yaw cmd : Scope
      settings: YMin=-60  YMax=60  SaveName=ScopeData10
  yaw_ref : Scope
      settings: TimeRange=39.996  YMin=-190  YMax=190  SaveName=ScopeData8
  z_ref : Scope
      settings: TimeRange=40  YMin=-21  YMax=1  SaveName=ScopeData5
  wires:
  bias/1 -> Bus Creator/4  "bias"
  Bus Selector8/1 -> "rad -> deg3"/1
  Bus Selector6/1 -> "rad -> deg2"/1
  Bus Selector5/1 -> "rad -> deg1"/1
  Bus Selector7/1 -> thrust cmd/1
  Bus Selector4/1 -> "rad -> deg"/1
  Bus Selector3/1 -> z_ref/1
  Bus Selector2/1 -> y_ref/1
  Bus Selector1/1 -> x_ref/1
  Bus Creator/1 -> Bus Selector8/1, Bus Selector7/1, Bus Selector6/1, Bus Selector5/1, Bus Selector4/1, Bus Selector3/1, Bus Selector2/1, Bus Selector1/1, Bus Selector10/1, Bus Selector9/1  "mega_bus"
  cmd/1 -> Bus Creator/3  "cmd"
  ref/1 -> Bus Creator/2  "ref"
  odometry/1 -> Bus Creator/1  "odometry"
  "rad -> deg3"/1 -> yaw cmd/1
  "rad -> deg2"/1 -> pitch cmd/1
  "rad -> deg1"/1 -> roll cmd/1
  "rad -> deg"/1 -> yaw_ref/1
  Bus Selector10/1 -> To File1/1
  Bus Selector9/1 -> To File/1

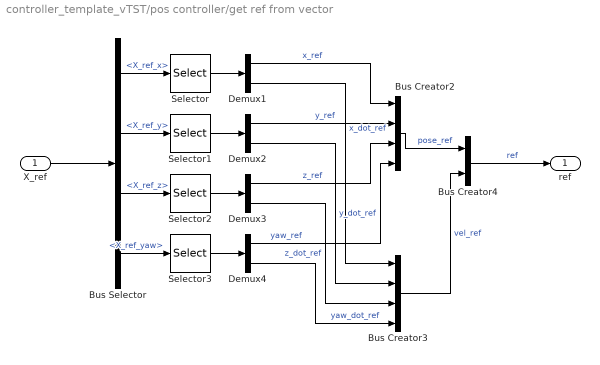
== system controller_template_vTST/pos controller/get ref from vector ==
  X_ref : Inport
  Bus Creator2 : BusCreator
  Bus Creator3 : BusCreator
  Bus Creator4 : BusCreator  Inputs=2
  Bus Selector : BusSelector  OutputSignals=X_ref_x,X_ref_y,X_ref_z,X_ref_yaw
  Demux{1..4} (4 alike) : Demux  Outputs=2
  Selector{,1..3} (4 alike) : Selector  IndexOptions=Index vector (dialog)  Indices=[1 2]  OutputSizes=1
  ref : Outport
  wires:
  X_ref/1 -> Bus Selector/1
  Bus Selector/1 -> Selector/1  "<X_ref_x>"
  Bus Selector/4 -> Selector3/1  "<X_ref_yaw>"
  Bus Selector/3 -> Selector2/1  "<X_ref_z>"
  Bus Selector/2 -> Selector1/1  "<X_ref_y>"
  Selector/1 -> Demux1/1
  Selector3/1 -> Demux4/1
  Selector2/1 -> Demux3/1
  Selector1/1 -> Demux2/1
  Bus Creator2/1 -> Bus Creator4/1  "pose_ref"
  Bus Creator3/1 -> Bus Creator4/2  "vel_ref"
  Bus Creator4/1 -> ref/1  "ref"
  Demux1/1 -> Bus Creator2/1  "x_ref"
  Demux2/1 -> Bus Creator2/2  "y_ref"
  Demux3/1 -> Bus Creator2/3  "z_ref"
  Demux4/1 -> Bus Creator2/4  "yaw_ref"
  Demux1/2 -> Bus Creator3/1  "x_dot_ref"
  Demux2/2 -> Bus Creator3/2  "y_dot_ref"
  Demux3/2 -> Bus Creator3/3  "z_dot_ref"
  Demux4/2 -> Bus Creator3/4  "yaw_dot_ref"

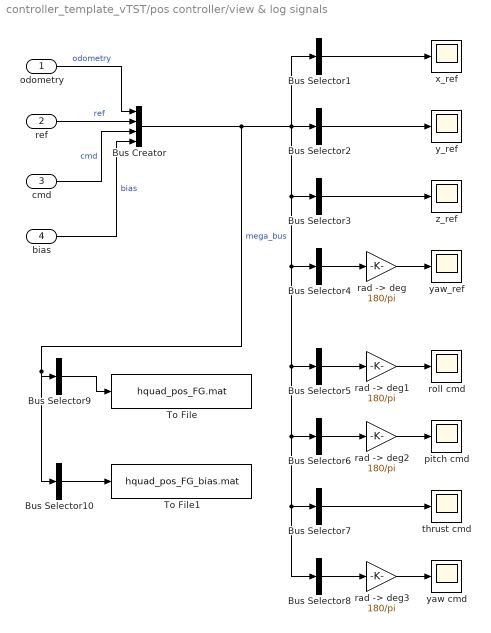
== system controller_template_vTST/pos controller/view & log signals ==
  odometry : Inport
  ref : Inport  Port=2
  cmd : Inport  Port=3
  bias : Inport  Port=4
  Bus Creator : BusCreator
  Bus Selector1 : BusSelector  OutputSignals=odometry.pos.x,odometry.vel.x_dot,ref.pose_ref.x_ref,ref.vel_ref.x_dot_ref  OutputAsBus=on
  Bus Selector10 : BusSelector  OutputSignals=bias.pitch_bias,bias.roll_bias,bias.thrust_bias,bias.yaw_rate_bias  OutputAsBus=on
  Bus Selector2 : BusSelector  OutputSignals=odometry.pos.y,odometry.vel.y_dot,ref.pose_ref.y_ref,ref.vel_ref.y_dot_ref  OutputAsBus=on
  Bus Selector3 : BusSelector  OutputSignals=odometry.pos.z,odometry.vel.z_dot,ref.pose_ref.z_ref,ref.vel_ref.z_dot_ref  OutputAsBus=on
  Bus Selector4 : BusSelector  OutputSignals=odometry.rpy.yaw,odometry.ang_vel.ang_vel_z,ref.pose_ref.yaw_ref,ref.vel_ref.yaw_dot_ref  OutputAsBus=on
  Bus Selector5 : BusSelector  OutputSignals=odometry.rpy.roll,odometry.ang_vel.ang_vel_x,cmd.roll_cmd  OutputAsBus=on
  Bus Selector6 : BusSelector  OutputSignals=odometry.rpy.pitch,odometry.ang_vel.ang_vel_y,cmd.pitch_cmd  OutputAsBus=on
  Bus Selector7 : BusSelector  OutputSignals=odometry.pos.z,ref.pose_ref.z_ref,cmd.thrust_cmd  OutputAsBus=on
  Bus Selector8 : BusSelector  OutputSignals=odometry.rpy.yaw,odometry.ang_vel.ang_vel_z,cmd.yaw_rate_cmd  OutputAsBus=on
  Bus Selector9 : BusSelector  OutputSignals=odometry.pos.x,odometry.vel.x_dot,odometry.rpy.pitch,ref.pose_ref.x_ref,cmd.pitch_cmd,odometry.pos.y,odometry.vel.y_dot,odometry.rpy.roll,ref.pose_ref.y_ref,cmd.roll_cmd,odometry.pos.z,odometry.vel.z_dot,ref.pose_ref.z_ref,cmd.thrust_cmd,odometry.rpy.yaw,odometry.ang_vel.ang_vel_z,ref.pose_ref.yaw_ref,cmd.yaw_rate_cmd  OutputAsBus=on
  To File : ToFile  Filename=hquad_pos_FG.mat  MatrixName=hquad_pos_FG
  To File1 : ToFile  Filename=hquad_pos_FG_bias.mat  MatrixName=hquad_pos_FG_bias
  pitch cmd : Scope
      settings: YMin=-15  YMax=15  SaveName=ScopeData2
  rad -> deg{,1..3} (4 alike) : Gain  Gain=180/pi
  roll cmd : Scope
      settings: YMin=-100  YMax=100
  thrust cmd : Scope
      settings: YMin=-3  YMax=3  SaveName=ScopeData11
  x_ref : Scope
      settings: YMin=-1.5  YMax=1.5  SaveName=ScopeData3
  y_ref : Scope
      settings: TimeRange=40  YMin=-0.75  YMax=2.75
  yaw cmd : Scope
      settings: YMin=-60  YMax=60  SaveName=ScopeData10
  yaw_ref : Scope
      settings: TimeRange=39.996  YMin=-190  YMax=190  SaveName=ScopeData8
  z_ref : Scope
      settings: TimeRange=40  YMin=-21  YMax=1  SaveName=ScopeData5
  wires:
  bias/1 -> Bus Creator/4  "bias"
  Bus Selector8/1 -> "rad -> deg3"/1
  Bus Selector6/1 -> "rad -> deg2"/1
  Bus Selector5/1 -> "rad -> deg1"/1
  Bus Selector7/1 -> thrust cmd/1
  Bus Selector4/1 -> "rad -> deg"/1
  Bus Selector3/1 -> z_ref/1
  Bus Selector2/1 -> y_ref/1
  Bus Selector1/1 -> x_ref/1
  Bus Creator/1 -> Bus Selector8/1, Bus Selector7/1, Bus Selector6/1, Bus Selector5/1, Bus Selector4/1, Bus Selector3/1, Bus Selector2/1, Bus Selector1/1, Bus Selector10/1, Bus Selector9/1  "mega_bus"
  cmd/1 -> Bus Creator/3  "cmd"
  ref/1 -> Bus Creator/2  "ref"
  odometry/1 -> Bus Creator/1  "odometry"
  "rad -> deg3"/1 -> yaw cmd/1
  "rad -> deg2"/1 -> pitch cmd/1
  "rad -> deg1"/1 -> roll cmd/1
  "rad -> deg"/1 -> yaw_ref/1
  Bus Selector10/1 -> To File1/1
  Bus Selector9/1 -> To File/1

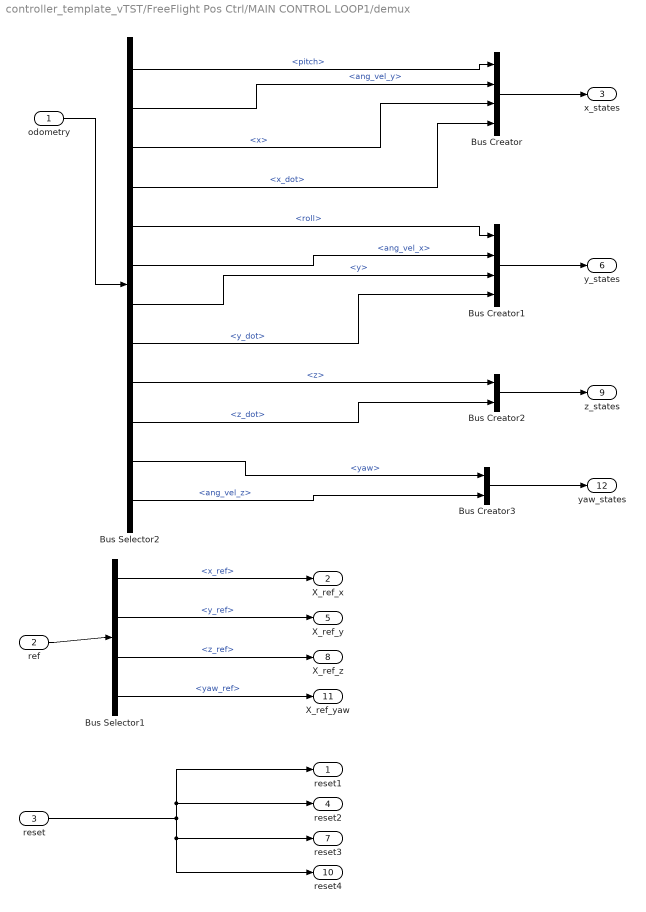
== system controller_template_vTST/FreeFlight Pos Ctrl/MAIN CONTROL LOOP1/demux ==
  odometry : Inport
  ref : Inport  Port=2
  reset : Inport  Port=3
  Bus Creator : BusCreator
  Bus Creator1 : BusCreator
  Bus Creator2 : BusCreator  Inputs=2
  Bus Creator3 : BusCreator  Inputs=2
  Bus Selector1 : BusSelector  OutputSignals=pose_ref.x_ref,pose_ref.y_ref,pose_ref.z_ref,pose_ref.yaw_ref
  Bus Selector2 : BusSelector  OutputSignals=rpy.pitch,ang_vel.ang_vel_y,pos.x,vel.x_dot,rpy.roll,ang_vel.ang_vel_x,pos.y,vel.y_dot,pos.z,vel.z_dot,rpy.yaw,ang_vel.ang_vel_z
  reset1 : Outport
  X_ref_x : Outport  Port=2
  x_states : Outport  Port=3
  reset2 : Outport  Port=4
  X_ref_y : Outport  Port=5
  y_states : Outport  Port=6
  reset3 : Outport  Port=7
  X_ref_z : Outport  Port=8
  z_states : Outport  Port=9
  reset4 : Outport  Port=10
  X_ref_yaw : Outport  Port=11
  yaw_states : Outport  Port=12
  wires:
  Bus Selector1/4 -> X_ref_yaw/1  "<yaw_ref>"
  Bus Selector1/3 -> X_ref_z/1  "<z_ref>"
  odometry/1 -> Bus Selector2/1
  ref/1 -> Bus Selector1/1
  Bus Selector1/1 -> X_ref_x/1  "<x_ref>"
  Bus Selector1/2 -> X_ref_y/1  "<y_ref>"
  reset/1 -> reset3/1, reset4/1, reset2/1, reset1/1
  Bus Selector2/1 -> Bus Creator/1  "<pitch>"
  Bus Selector2/2 -> Bus Creator/2  "<ang_vel_y>"
  Bus Selector2/3 -> Bus Creator/3  "<x>"
  Bus Selector2/4 -> Bus Creator/4  "<x_dot>"
  Bus Creator1/1 -> y_states/1
  Bus Selector2/5 -> Bus Creator1/1  "<roll>"
  Bus Selector2/6 -> Bus Creator1/2  "<ang_vel_x>"
  Bus Selector2/7 -> Bus Creator1/3  "<y>"
  Bus Selector2/8 -> Bus Creator1/4  "<y_dot>"
  Bus Selector2/9 -> Bus Creator2/1  "<z>"
  Bus Selector2/10 -> Bus Creator2/2  "<z_dot>"
  Bus Selector2/12 -> Bus Creator3/2  "<ang_vel_z>"
  Bus Selector2/11 -> Bus Creator3/1  "<yaw>"
  Bus Creator2/1 -> z_states/1
  Bus Creator3/1 -> yaw_states/1
  Bus Creator/1 -> x_states/1

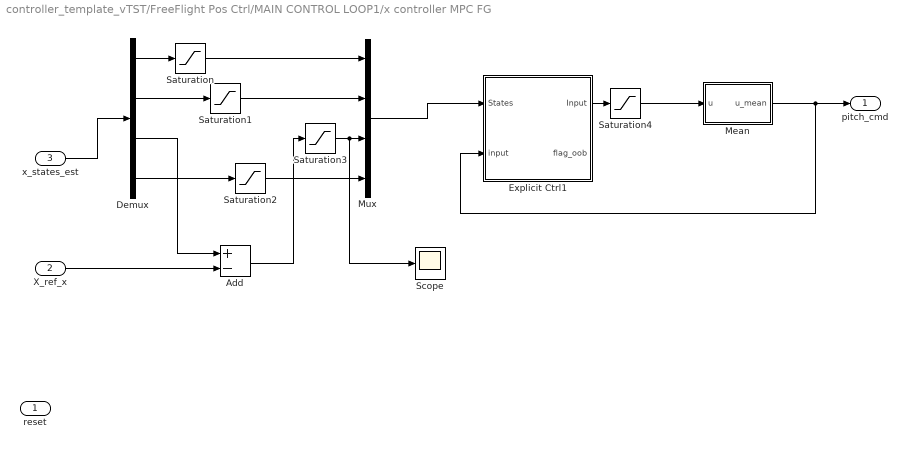
== system controller_template_vTST/FreeFlight Pos Ctrl/MAIN CONTROL LOOP1/x controller MPC FG   ==
  reset : Inport  PortDimensions=1
  "X_ref_x  " : Inport  Port=2
  "x_states_est  " : Inport  Port=3
  Add : Sum  Inputs=+-
  Demux : Demux
  Explicit Ctrl1 : Subsystem
  Mean : Subsystem
  Mux : Mux
  Saturation : Saturate  UpperLimit=0.2094  LowerLimit=-0.2094
  Saturation1 : Saturate  UpperLimit=2  LowerLimit=-2
  Saturation2 : Saturate  UpperLimit=1  LowerLimit=-1
  Saturation3 : Saturate  UpperLimit=1  LowerLimit=-1
  Saturation4 : Saturate  UpperLimit=0.2094  LowerLimit=-0.2094
  Scope : Scope
      settings: SaveName=ScopeData11
  "pitch_cmd   " : Outport  PortDimensions=1
  wires:
  "X_ref_x  "/1 -> Add/2
  Demux/1 -> Saturation/1
  Demux/2 -> Saturation1/1
  Demux/3 -> Add/1
  Add/1 -> Saturation3/1
  Mux/1 -> Explicit Ctrl1/1(States)
  "x_states_est  "/1 -> Demux/1
  Saturation/1 -> Mux/1
  Saturation1/1 -> Mux/2
  Saturation2/1 -> Mux/4
  Saturation3/1 -> Scope/1, Mux/3
  Explicit Ctrl1/1(Input) -> Saturation4/1
  Mean/1(u_mean) -> "pitch_cmd   "/1, Explicit Ctrl1/2(input)
  Saturation4/1 -> Mean/1(u)
  Demux/4 -> Saturation2/1

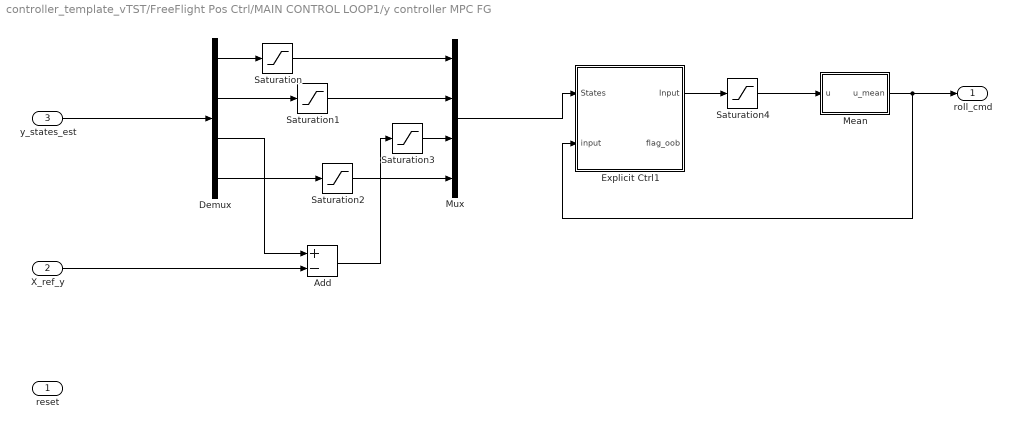
== system controller_template_vTST/FreeFlight Pos Ctrl/MAIN CONTROL LOOP1/y controller MPC FG ==
  reset : Inport  PortDimensions=1
  "X_ref_y  " : Inport  Port=2
  "y_states_est  " : Inport  Port=3
  Add : Sum  Inputs=+-
  Demux : Demux
  Explicit Ctrl1 : Subsystem
  Mean : Subsystem
  Mux : Mux
  Saturation : Saturate  UpperLimit=0.2094  LowerLimit=-0.2094
  Saturation1 : Saturate  UpperLimit=2  LowerLimit=-2
  Saturation2 : Saturate  UpperLimit=1  LowerLimit=-1
  Saturation3 : Saturate  UpperLimit=1  LowerLimit=-1
  Saturation4 : Saturate  UpperLimit=0.2094  LowerLimit=-0.2094
  roll_cmd : Outport  PortDimensions=1
  wires:
  Explicit Ctrl1/1(Input) -> Saturation4/1
  "X_ref_y  "/1 -> Add/2
  Demux/1 -> Saturation/1
  Demux/2 -> Saturation1/1
  Demux/3 -> Add/1
  Add/1 -> Saturation3/1
  Demux/4 -> Saturation2/1
  Mux/1 -> Explicit Ctrl1/1(States)
  "y_states_est  "/1 -> Demux/1
  Saturation/1 -> Mux/1
  Saturation1/1 -> Mux/2
  Saturation2/1 -> Mux/4
  Saturation3/1 -> Mux/3
  Mean/1(u_mean) -> roll_cmd/1, Explicit Ctrl1/2(input)
  Saturation4/1 -> Mean/1(u)

== system controller_template_vTST/FreeFlight Pos Ctrl/MAIN CONTROL LOOP1/yaw controller MPC FG ==
  reset : Inport  PortDimensions=1
  X_ref_yaw : Inport  Port=2
  "yaw_states_est  " : Inport  Port=3
  Add : Sum  Inputs=+-
  Demux : Demux  Outputs=2
  Explicit Ctrl1 : Subsystem
  Mean : Subsystem
  Saturation : Saturate  UpperLimit=pi  LowerLimit=-pi
  Saturation1 : Saturate  UpperLimit=pi  LowerLimit=-pi
  yaw_rate_cmd : Outport  PortDimensions=1
  wires:
  X_ref_yaw/1 -> Add/2
  "yaw_states_est  "/1 -> Demux/1
  Demux/1 -> Add/1
  Add/1 -> Saturation/1
  Saturation/1 -> Explicit Ctrl1/1(States)
  Explicit Ctrl1/1(Input) -> Saturation1/1
  Mean/1(u_mean) -> yaw_rate_cmd/1, Explicit Ctrl1/2(input)
  Saturation1/1 -> Mean/1(u)

== system controller_template_vTST/FreeFlight Pos Ctrl/MAIN CONTROL LOOP1/z controller MPC FG ==
  reset : Inport  PortDimensions=1
  X_ref_z : Inport  Port=2
  "z_states_est  " : Inport  Port=3
  Add : Sum  Inputs=+-
  Demux : Demux  Outputs=2
  Explicit Ctrl1 : Subsystem
  Mean : Subsystem
  Mux : Mux  Inputs=2
  Saturation : Saturate  UpperLimit=1  LowerLimit=-1
  Saturation1 : Saturate  UpperLimit=1  LowerLimit=-1
  Saturation2 : Saturate  UpperLimit=1  LowerLimit=-1
  Scope : Scope
      settings: SaveName=ScopeData2
  thrust_cmd : Outport  PortDimensions=1
  wires:
  "z_states_est  "/1 -> Demux/1
  Demux/2 -> Saturation/1
  Demux/1 -> Add/1
  X_ref_z/1 -> Add/2
  Add/1 -> Saturation1/1
  Mux/1 -> Explicit Ctrl1/1(States), Scope/1
  Saturation/1 -> Mux/2
  Saturation1/1 -> Mux/1
  Explicit Ctrl1/1(Input) -> Saturation2/1
  Mean/1(u_mean) -> thrust_cmd/1
  Saturation2/1 -> Mean/1(u)

== system controller_template_vTST/FreeFlight Pos Ctrl/MAIN CONTROL LOOP1/x controller MPC FG  /Explicit Ctrl1 ==
  States : Inport
  input : Inport  Port=2
  Constant : Constant  Value=Hn_XdirFF
  Constant1 : Constant  Value=Kn_XdirFF
  Constant2 : Constant  Value=Fi_XdirFF
  Constant3 : Constant  Value=Gi_XdirFF
  Constant4 : Constant  Value=Nc_XdirFF
  Ctrl_Xdir : MATLAB Function  TreatAsAtomicUnit=on
  PitchPropagate : Subsystem
  Rate Transition : RateTransition  OutPortSampleTime=0.08
  Rate Transition1 : RateTransition  OutPortSampleTime=0.08
  Unit Delay2 : UnitDelay  SampleTime=-1
  Input : Outport
  flag_oob : Outport  Port=2
  wires:
  Ctrl_Xdir/2(flag_oob) -> flag_oob/1
  Ctrl_Xdir/1(U) -> Input/1
  Constant4/1 -> Ctrl_Xdir/6(Nc)
  Constant3/1 -> Ctrl_Xdir/5(Gi)
  Constant2/1 -> Ctrl_Xdir/4(Fi)
  Constant1/1 -> Ctrl_Xdir/3(Kn)
  Constant/1 -> Ctrl_Xdir/2(Hn)
  States/1 -> Rate Transition/1
  Unit Delay2/1 -> PitchPropagate/1(uprev)
  Rate Transition/1 -> PitchPropagate/2(x)
  PitchPropagate/1(Out1) -> Ctrl_Xdir/1(X)
  input/1 -> Rate Transition1/1
  Rate Transition1/1 -> Unit Delay2/1

== system controller_template_vTST/FreeFlight Pos Ctrl/MAIN CONTROL LOOP1/x controller MPC FG  /Mean ==
  u : Inport
  Gain : Gain  Gain=.33333
  Sum : Sum  Inputs=|++
  Sum1 : Sum  Inputs=|++
  Unit Delay : UnitDelay  SampleTime=-1
  Unit Delay1 : UnitDelay  SampleTime=-1
  Unit Delay2 : UnitDelay  SampleTime=-1
  u_mean : Outport
  wires:
  u/1 -> Sum/1
  Sum/1 -> Gain/1
  Gain/1 -> u_mean/1, Unit Delay1/1, Unit Delay2/1
  Unit Delay1/1 -> Unit Delay/1
  Unit Delay/1 -> Sum1/2
  Sum1/1 -> Sum/2
  Unit Delay2/1 -> Sum1/1

== system controller_template_vTST/FreeFlight Pos Ctrl/MAIN CONTROL LOOP1/y controller MPC FG/Explicit Ctrl1 ==
  States : Inport
  input : Inport  Port=2
  Constant : Constant  Value=Hn_Ydir
  Constant1 : Constant  Value=Kn_Ydir
  Constant2 : Constant  Value=Fi_Ydir
  Constant3 : Constant  Value=Gi_Ydir
  Constant4 : Constant  Value=Nc_Ydir
  Ctrl_Xdir : MATLAB Function  TreatAsAtomicUnit=on
  Rate Transition : RateTransition  OutPortSampleTime=0.08
  Rate Transition1 : RateTransition  OutPortSampleTime=0.08
  RollPropagate : Subsystem
  Unit Delay2 : UnitDelay  SampleTime=-1
  Input : Outport
  flag_oob : Outport  Port=2
  wires:
  Ctrl_Xdir/2(flag_oob) -> flag_oob/1
  Ctrl_Xdir/1(U) -> Input/1
  Constant4/1 -> Ctrl_Xdir/6(Nc)
  Constant3/1 -> Ctrl_Xdir/5(Gi)
  Constant2/1 -> Ctrl_Xdir/4(Fi)
  Constant1/1 -> Ctrl_Xdir/3(Kn)
  Constant/1 -> Ctrl_Xdir/2(Hn)
  States/1 -> Rate Transition/1
  Unit Delay2/1 -> RollPropagate/1(uprev)
  Rate Transition/1 -> RollPropagate/2(x)
  RollPropagate/1(Out1) -> Ctrl_Xdir/1(X)
  input/1 -> Rate Transition1/1
  Rate Transition1/1 -> Unit Delay2/1

== system controller_template_vTST/FreeFlight Pos Ctrl/MAIN CONTROL LOOP1/y controller MPC FG/Mean ==
  u : Inport
  Gain : Gain  Gain=.33333
  Sum : Sum  Inputs=|++
  Sum1 : Sum  Inputs=|++
  Unit Delay : UnitDelay  SampleTime=-1
  Unit Delay1 : UnitDelay  SampleTime=-1
  Unit Delay2 : UnitDelay  SampleTime=-1
  u_mean : Outport
  wires:
  u/1 -> Sum/1
  Sum/1 -> Gain/1
  Gain/1 -> u_mean/1, Unit Delay1/1, Unit Delay2/1
  Unit Delay1/1 -> Unit Delay/1
  Unit Delay/1 -> Sum1/2
  Sum1/1 -> Sum/2
  Unit Delay2/1 -> Sum1/1

== system controller_template_vTST/FreeFlight Pos Ctrl/MAIN CONTROL LOOP1/yaw controller MPC FG/Explicit Ctrl1 ==
  States : Inport
  input : Inport  Port=2
  Constant : Constant  Value=Hn_Yaw
  Constant1 : Constant  Value=Kn_Yaw
  Constant2 : Constant  Value=Fi_Yaw
  Constant3 : Constant  Value=Gi_Yaw
  Constant4 : Constant  Value=Nc_Yaw
  Ctrl_Xdir : MATLAB Function  TreatAsAtomicUnit=on
  Rate Transition : RateTransition  OutPortSampleTime=0.08
  Rate Transition1 : RateTransition  OutPortSampleTime=0.08
  Unit Delay2 : UnitDelay  SampleTime=-1
  YawPropagate : Subsystem
  Input : Outport
  flag_oob : Outport  Port=2
  wires:
  Ctrl_Xdir/2(flag_oob) -> flag_oob/1
  Ctrl_Xdir/1(U) -> Input/1
  Constant4/1 -> Ctrl_Xdir/6(Nc)
  Constant3/1 -> Ctrl_Xdir/5(Gi)
  Constant2/1 -> Ctrl_Xdir/4(Fi)
  Constant1/1 -> Ctrl_Xdir/3(Kn)
  Constant/1 -> Ctrl_Xdir/2(Hn)
  States/1 -> Rate Transition/1
  Unit Delay2/1 -> YawPropagate/1(uprev)
  Rate Transition/1 -> YawPropagate/2(x)
  YawPropagate/1(Out1) -> Ctrl_Xdir/1(X)
  input/1 -> Rate Transition1/1
  Rate Transition1/1 -> Unit Delay2/1

== system controller_template_vTST/FreeFlight Pos Ctrl/MAIN CONTROL LOOP1/yaw controller MPC FG/Mean ==
  u : Inport
  Gain : Gain  Gain=.33333
  Sum : Sum  Inputs=|++
  Sum1 : Sum  Inputs=|++
  Unit Delay : UnitDelay  SampleTime=-1
  Unit Delay1 : UnitDelay  SampleTime=-1
  Unit Delay2 : UnitDelay  SampleTime=-1
  u_mean : Outport
  wires:
  u/1 -> Sum/1
  Sum/1 -> Gain/1
  Gain/1 -> u_mean/1, Unit Delay1/1, Unit Delay2/1
  Unit Delay1/1 -> Unit Delay/1
  Unit Delay/1 -> Sum1/2
  Sum1/1 -> Sum/2
  Unit Delay2/1 -> Sum1/1

== system controller_template_vTST/FreeFlight Pos Ctrl/MAIN CONTROL LOOP1/z controller MPC FG/Explicit Ctrl1 ==
  States : Inport
  Constant : Constant  Value=Hn_Zdir
  Constant1 : Constant  Value=Kn_Zdir
  Constant2 : Constant  Value=Fi_Zdir
  Constant3 : Constant  Value=Gi_Zdir
  Constant4 : Constant  Value=Nc_Zdir
  Ctrl_Xdir : MATLAB Function  TreatAsAtomicUnit=on
  Rate Transition : RateTransition  OutPortSampleTime=0.08
  Input : Outport
  flag_oob : Outport  Port=2
  wires:
  Ctrl_Xdir/2(flag_oob) -> flag_oob/1
  Rate Transition/1 -> Ctrl_Xdir/1(X)
  Ctrl_Xdir/1(U) -> Input/1
  Constant4/1 -> Ctrl_Xdir/6(Nc)
  Constant3/1 -> Ctrl_Xdir/5(Gi)
  Constant2/1 -> Ctrl_Xdir/4(Fi)
  Constant1/1 -> Ctrl_Xdir/3(Kn)
  Constant/1 -> Ctrl_Xdir/2(Hn)
  States/1 -> Rate Transition/1

== system controller_template_vTST/FreeFlight Pos Ctrl/MAIN CONTROL LOOP1/z controller MPC FG/Mean ==
  u : Inport
  Gain : Gain  Gain=.33333
  Sum : Sum  Inputs=|++
  Sum1 : Sum  Inputs=|++
  Unit Delay : UnitDelay  SampleTime=-1
  Unit Delay1 : UnitDelay  SampleTime=-1
  Unit Delay2 : UnitDelay  SampleTime=-1
  u_mean : Outport
  wires:
  u/1 -> Sum/1
  Sum/1 -> Gain/1
  Gain/1 -> u_mean/1, Unit Delay1/1, Unit Delay2/1
  Unit Delay1/1 -> Unit Delay/1
  Unit Delay/1 -> Sum1/2
  Sum1/1 -> Sum/2
  Unit Delay2/1 -> Sum1/1

== system controller_template_vTST/FreeFlight Pos Ctrl/MAIN CONTROL LOOP1/x controller MPC FG  /Explicit Ctrl1/PitchPropagate ==
  uprev : Inport
  x : Inport  Port=2
  Constant : Constant  Value=Aff_pitch
  Constant1 : Constant  Value=Bff_pitch
  MATLAB Function : MATLAB Function  TreatAsAtomicUnit=on
  Out1 : Outport
  wires:
  MATLAB Function/1(y) -> Out1/1
  x/1 -> MATLAB Function/1(x)
  uprev/1 -> MATLAB Function/4(u)
  Constant/1 -> MATLAB Function/2(A)
  Constant1/1 -> MATLAB Function/3(B)

== system controller_template_vTST/FreeFlight Pos Ctrl/MAIN CONTROL LOOP1/y controller MPC FG/Explicit Ctrl1/RollPropagate ==
  uprev : Inport
  x : Inport  Port=2
  Constant : Constant  Value=Aff_roll
  Constant1 : Constant  Value=Bff_roll
  MATLAB Function : MATLAB Function  TreatAsAtomicUnit=on
  Out1 : Outport
  wires:
  MATLAB Function/1(y) -> Out1/1
  x/1 -> MATLAB Function/1(x)
  uprev/1 -> MATLAB Function/4(u)
  Constant/1 -> MATLAB Function/2(A)
  Constant1/1 -> MATLAB Function/3(B)

== system controller_template_vTST/FreeFlight Pos Ctrl/MAIN CONTROL LOOP1/yaw controller MPC FG/Explicit Ctrl1/YawPropagate ==
  uprev : Inport
  x : Inport  Port=2
  Constant : Constant  Value=Aff_yaw
  Constant1 : Constant  Value=Bff_yaw
  MATLAB Function : MATLAB Function  TreatAsAtomicUnit=on
  Out1 : Outport
  wires:
  MATLAB Function/1(y) -> Out1/1
  x/1 -> MATLAB Function/1(x)
  uprev/1 -> MATLAB Function/4(u)
  Constant/1 -> MATLAB Function/2(A)
  Constant1/1 -> MATLAB Function/3(B)

== matlab function FreeFlight Pos Ctrl/MAIN CONTROL LOOP1/x controller MPC FG /Explicit Ctrl1/Ctrl_Xdir ==
  data: X input double; U output double; Hn input double; Kn input double; Fi input double; Gi input double; Nc input double; flag_oob output double
function [U,flag_oob] = OptimalMPCInput(X,Hn,Kn,Fi,Gi,Nc)

tolerance = 1;
nr  = size(Nc,1);
MPT_ABSTOL = 1e-8;
minreg = 0;
X = round(10000*X)/10000;

flag_oob = 0;
%maxSize = max(Nc);

Hi = zeros(100,4);
Ki = zeros(100,1);

% Find the proper region
abspos = 1;
for ireg = 1:nr
    sumViol = 0;
    isinside = 1;
    

  %  Hi(1:Nc(ireg),1:4) = Hn(abspos:(abspos+Nc(ireg)-1),1:4);
    for i = 1:Nc(ireg)
        for j = 1:4
            Hi(i,j) = Hn(abspos + i - 1,j);
        end
    end
    
%    Ki(1:Nc(ireg),1) = Kn(abspos:(abspos+Nc(ireg)-1),1);
    for i = 1:Nc(ireg)
        Ki(i,1) = Kn(abspos + i - 1,1);
    end
    abspos = abspos + Nc(ireg);
    
    F = Fi(ireg,:);
    G = Gi(ireg,:);
    
    nc = Nc(ireg);
    
    for ic = 1:nc
        hx = Hi(ic,:)*X;
        if ((hx - Ki(ic)) > MPT_ABSTOL)
            isinside = 0;
            sumViol = sumViol + (hx - Ki(ic));
        end
    end
    
    if (sumViol < tolerance)
        tolerance = sumViol;
        minreg = ireg;
    end
    % extract the right control law
    if (isinside == 1)
        U = F*X + G;
        return
    end
end
F = Fi(minreg,:);
G = Gi(minreg,:);
U = F*X + G;
flag_oob = 1;
%U = U_prev;
return
